simulink model "untitled"  (R2016b)
settings: Solver=FixedStepAuto  StartTime=0.0  StopTime=10.0  FixedStep=0.002  RelTol=1e-3
libraries: simulink x1
settings Model: Creator=lucadelaat  LastModifiedBy=lucadelaat

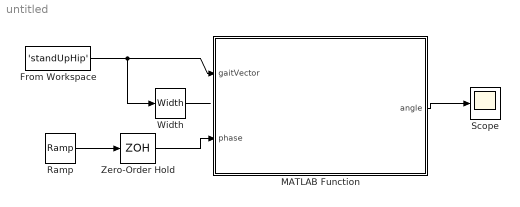
== system untitled ==
  From Workspace : FromWorkspace  VariableName='standUpHip'  SampleTime=0  Interpolate=off  OutputAfterFinalValue=Holding final value
  MATLAB Function : MATLAB Function  TreatAsAtomicUnit=on
  Ramp : simulink/Sources/Ramp  slope=1  start=0  X0=0
  Scope : Scope
  Width : Width
  Zero-Order Hold : ZeroOrderHold  SampleTime=-1
  wires:
  Ramp/1 -> Zero-Order Hold/1
  From Workspace/1 -> Width/1, MATLAB Function/1(gaitVector)
  MATLAB Function/1(angle) -> Scope/1
  Zero-Order Hold/1 -> MATLAB Function/2(phase)
  Width/1 -> ?

== matlab function untitled/MATLAB Function ==
  data: gaitVector input; angle output; phase input
function angle  = lookup_table(gaitVector, phase)
% wrapper for lookup_table
[angle] = lookup_table(gaitVector, phase);
end
